simulink model "simulate_fixed_complex_trajectories"  (R2021a)
settings: Solver=VariableStepAuto  StartTime=0.0  StopTime=100  RelTol=1e-3
PreLoadFcn:
  | set_param_fixed_complex;
undefined symbols (not defined in the file or in its folder): ParamFixComplex, ParamFixLine, ParamFixOrb
settings Model: Creator=diogo  LastModifiedBy=Nunes
settings SolverCC: AlgebraicLoopSolver=TrustRegion
settings DebuggingCC: SFMachineParentedDataDiag=warning

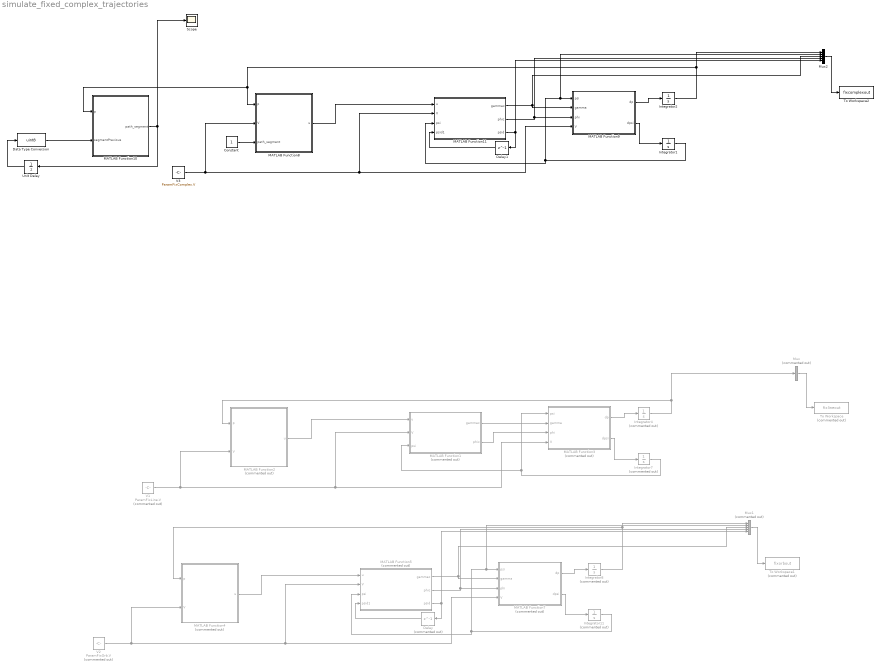
== system simulate_fixed_complex_trajectories ==
  Constant : Constant  OutDataTypeStr=uint8
  Data Type Conversion : DataTypeConversion  OutDataTypeStr=uint8
  Delay : Delay  Commented=on  DelayLength=1  InitialCondition=0
  Delay1 : Delay  DelayLength=1  InitialCondition=0
  Integrator1 : Integrator  InitialCondition=ParamFixComplex.psi0
  Integrator11 : Integrator  Commented=on  InitialCondition=ParamFixOrb.psi0
  Integrator2 : Integrator  InitialCondition=ParamFixComplex.p0
  Integrator4 : Integrator  Commented=on  InitialCondition=ParamFixLine.p0
  Integrator7 : Integrator  Commented=on  InitialCondition=ParamFixLine.psi0
  Integrator8 : Integrator  Commented=on  InitialCondition=ParamFixOrb.p0
  MATLAB Function1 : MATLAB Function  Commented=on  TreatAsAtomicUnit=on
  MATLAB Function10 : MATLAB Function  TreatAsAtomicUnit=on
  MATLAB Function11 : MATLAB Function  TreatAsAtomicUnit=on
  MATLAB Function2 : MATLAB Function  Commented=on  TreatAsAtomicUnit=on
  MATLAB Function3 : MATLAB Function  Commented=on  TreatAsAtomicUnit=on
  MATLAB Function4 : MATLAB Function  Commented=on  TreatAsAtomicUnit=on
  MATLAB Function5 : MATLAB Function  Commented=on  TreatAsAtomicUnit=on
  MATLAB Function7 : MATLAB Function  Commented=on  TreatAsAtomicUnit=on
  MATLAB Function8 : MATLAB Function  TreatAsAtomicUnit=on
  MATLAB Function9 : MATLAB Function  TreatAsAtomicUnit=on
  Mux : Mux  Commented=on  Inputs=1
  Mux1 : Mux  Commented=on  Inputs=5
  Mux2 : Mux  Inputs=5
  Scope : Scope
  To Workspace : ToWorkspace  Commented=on  VariableName=fixlineout  SaveFormat=Timeseries  SampleTime=-1
  To Workspace1 : ToWorkspace  Commented=on  VariableName=fixorbout  SaveFormat=Timeseries  SampleTime=-1
  To Workspace2 : ToWorkspace  VariableName=fixcomplexout  SaveFormat=Timeseries  SampleTime=-1
  Unit Delay : UnitDelay  InitialCondition=1  SampleTime=-1  HasFrameUpgradeWarning=on
  V1 : Constant  Commented=on  Value=ParamFixLine.V
  V2 : Constant  Commented=on  Value=ParamFixOrb.V
  V3 : Constant  Value=ParamFixComplex.V
  wires:
  MATLAB Function3/1(dp) -> Integrator4/1
  MATLAB Function3/2(dpsi) -> Integrator7/1
  Integrator7/1 -> MATLAB Function1/3(psi), MATLAB Function3/1(psi)
  MATLAB Function1/2(phic) -> MATLAB Function3/3(phi)
  MATLAB Function1/1(gammac) -> MATLAB Function3/2(gamma)
  V1/1 -> MATLAB Function2/2(V), MATLAB Function1/2(V), MATLAB Function3/4(V)
  Integrator4/1 -> MATLAB Function2/1(p), Mux/1
  MATLAB Function2/1(u) -> MATLAB Function1/1(u)
  Mux/1 -> To Workspace/1
  MATLAB Function5/2(phic) -> Mux1/4, MATLAB Function7/3(phi)
  MATLAB Function7/1(dp) -> Integrator8/1
  V2/1 -> MATLAB Function4/2(V), MATLAB Function5/2(V), MATLAB Function7/4(V)
  MATLAB Function7/2(dpsi) -> Integrator11/1
  Integrator11/1 -> Mux1/2, MATLAB Function7/1(psi), MATLAB Function5/3(psi)
  Mux1/1 -> To Workspace1/1
  MATLAB Function5/1(gammac) -> Mux1/3, MATLAB Function7/2(gamma)
  Integrator8/1 -> MATLAB Function4/1(p), Mux1/1
  MATLAB Function4/1(u) -> MATLAB Function5/1(u)
  MATLAB Function5/3(psid) -> Mux1/5, Delay/1
  Delay/1 -> MATLAB Function5/4(psid1)
  MATLAB Function11/3(psid) -> Mux2/5, Delay1/1
  Delay1/1 -> MATLAB Function11/4(psid1)
  V3/1 -> MATLAB Function8/2(V), MATLAB Function11/2(V), MATLAB Function9/4(V)
  Integrator2/1 -> Mux2/1, MATLAB Function8/1(p), MATLAB Function10/1(p)
  MATLAB Function11/1(gammac) -> Mux2/3, MATLAB Function9/2(gamma)
  Mux2/1 -> To Workspace2/1
  MATLAB Function8/1(u) -> MATLAB Function11/1(u)
  MATLAB Function9/1(dp) -> Integrator2/1
  MATLAB Function9/2(dpsi) -> Integrator1/1
  MATLAB Function11/2(phic) -> Mux2/4, MATLAB Function9/3(phi)
  Integrator1/1 -> MATLAB Function11/3(psi), Mux2/2, MATLAB Function9/1(psi)
  Unit Delay/1 -> Data Type Conversion/1
  Data Type Conversion/1 -> MATLAB Function10/2(segmentPrevious)
  MATLAB Function10/1(path_segment) -> Scope/1, Unit Delay/1
  Constant/1 -> MATLAB Function8/3(path_segment)

== matlab function simulate_fixed_complex_trajectories/MATLAB Function10 ==
  data: p input; path_segment output; ParamFixComplex parameter; segmentPrevious input
function path_segment   = complex_path_manager(p,  ParamFixComplex, segmentPrevious)
 
path_segment = segmentPrevious;

number_of_segments = size(ParamFixComplex.c0_l);
number_of_segments = number_of_segments(2);

if path_segment == number_of_segments
    
   % number_of_segments = cast(number_of_segments, "uint8");
    %segment = number_of_segments - 1;

    
    c_n = ParamFixComplex.c0_l(1, path_segment );   
    c_e = ParamFixComplex.c0_l(2,path_segment );
    c_d = ParamFixComplex.c0_l(3,path_segment);

else 
    
    c_n = ParamFixComplex.c0_l(1, path_segment + 1);   
    c_e = ParamFixComplex.c0_l(2,path_segment + 1);
    c_d = ParamFixComplex.c0_l(3,path_segment + 1);

end



distance_to_next_path = sqrt((c_n - p(1))^2 + (c_e - p(2))^2 + (c_d - p(3))^2);
proximity_radius = 10;


if distance_to_next_path < proximity_radius
    path_segment = path_segment + 1 ;

end







end


















% if distance_to_next_path < proximity_radius
%     segment = 2;

% %second line starting point
% c_n = ParamFixComplex.c0_l(1, segmentPrevious + 1);   
% c_e = ParamFixComplex.c0_l(2,segmentPrevious + 1);
% c_d = ParamFixComplex.c0_l(3,segmentPrevious + 1);
% 
% 
% distance_to_next_path = sqrt((c_n - p(1))^2 + (c_e - p(2))^2 + (c_d - p(3))^2);
% proximity_radius = 10;
% 
% 
% if distance_to_next_path < proximity_radius
%     segment = 2;
% 
% else 
%     segment = segmentPrevious;
% end
% 
% % path_segment = segment;

== matlab function simulate_fixed_complex_trajectories/MATLAB Function11 ==
  data: u input; V input; psi input; psid1 input; gammac output; phic output; ParamFixComplex parameter; psid output
function [  gammac, phic, psid] = path_following_controller(u, V, psi, psid1, ParamFixComplex)

gamma_limit = ParamFixComplex.gamma_limit;
phi_limit = ParamFixComplex.phi_limit;
kphi = ParamFixComplex.kphi;

gammac = -sat(asin(u(3)/V), gamma_limit);

psid = atan2(u(2),u(1));

while abs(psid - psid1) > 3*pi/2
    if((psid - psid1) > 3*pi/2) 
        psid = psid- 2*pi;
    elseif ((psid - psid1) < - 3*pi/2)
        psid = psid + 2*pi;
    end
end

if(abs(psid - psid1) > pi)
    xpto = 0;
end;

phic = sat(kphi*(psid - psi), phi_limit);

end

== matlab function simulate_fixed_complex_trajectories/MATLAB Function1 ==
  data: u input; V input; psi input; gammac output; phic output; ParamFixLine parameter
function [  gammac, phic] = path_following_controller(u, V, psi, ParamFixLine)


gamma_limit = ParamFixLine.gamma_limit;
phi_limit = ParamFixLine.phi_limit;
kphi = ParamFixLine.kphi;

gammac = -sat(asin(u(3)/V), gamma_limit);

psid = atan2(u(2),u(1));

phic = sat(kphi*(psid- psi), phi_limit);

end

== matlab function simulate_fixed_complex_trajectories/MATLAB Function2 ==
  data: p input; u output; V input; ParamFixLine parameter
function u  = straight_path_generator(p, V, ParamFixLine)


%Variables

psi_l = ParamFixLine.psi_l;  %desired heading angle
gamma_l = ParamFixLine.gamma_l; %desired flight path angle

c_n = ParamFixLine.c0(1);    %path starting point
c_e = ParamFixLine.c0(2);
c_d = ParamFixLine.c0(3);

r_n = p(1);    %position
r_e = p(2);
r_d = p(3);
r = [r_n; r_e; r_d];

cl = [c_n; c_e; c_d];

ql = [cos(psi_l)*cos(gamma_l) ; sin(psi_l)*cos(gamma_l) ; -sin(gamma_l) ];
%direction of line




n_lon = [ -sin(psi_l) ; cos(psi_l) ; 0 ]; 

n_lat = [-cos(psi_l)*sin(gamma_l) ; -sin(psi_l)*sin(gamma_l) ; -cos(gamma_l) ];

k1 = 1;
k2 = 1;

%u_line = k1*(n_lon*transpose(n_lon) +  n_lat*transpose(n_lat))*(r - cl) + k2*cross(n_lon,n_lat);
u_line = -k1*(n_lon*n_lon' +  n_lat*n_lat')*(r - cl) - k2*cross(n_lon,n_lat);

u = V*(u_line/norm(u_line));



end

== matlab function simulate_fixed_complex_trajectories/MATLAB Function3 ==
  data: psi input; gamma input; phi input; V input; dp output; dpsi output
function [dp, dpsi] = drone_model(psi,gamma,phi, V)
    
    %criar param para generalizar os valores
    
    %dp = [V*cos(psi)*cos(gamma); V*sin(psi)*cos(gamma); -V*sin(gamma)]
    
    dpn =V*cos(psi)*cos(gamma);
    dpe = V*sin(psi)*cos(gamma);
    dpd = -V*sin(gamma);
    dpsi =  (9.8/V)*tan(phi);
    
    dp = [dpn; dpe; dpd];
end

== matlab function simulate_fixed_complex_trajectories/MATLAB Function4 ==
  data: p input; u output; V input; ParamFixOrb parameter
function u  = orbit_path_generator(p, V, ParamFixOrb)


%Variables

 Rh = ParamFixOrb.Rh;
 lambda = ParamFixOrb.lambda;
 gamma_h = ParamFixOrb.gamma_h;
 psi_h = ParamFixOrb.psi_h;
 
k1 = ParamFixOrb.k1;
k2 = ParamFixOrb.k2;
 

ch = ParamFixOrb.ch;

c_n = ch(1);    %center of helix
c_e = ch(2);
c_d = ch(3);


 r_n = p(1);
 r_e = p(2);
 r_d = p(3);
 
 
%r0 = ch + [Rh*cos(psi_h) ; Rh*sin(psi_h) ; 0];

dalpha_cyl = transpose( [ 2*(r_n - c_n)/Rh ; 2*(r_e - c_e)/Rh ; 0 ] );

dalpha_pl = transpose( [ (tan(gamma_h)/lambda)*(-(r_e - c_e))/( (r_n - c_n)^2 + (r_e - c_e)^2 ) ; (tan(gamma_h)/lambda)*(r_n - c_e)/( (r_n - c_n)^2 + (r_e - c_e)^2 )  ; 1/Rh ] );


alpha_cyl = ( (r_n - c_n)/Rh )^2 + ( (r_e - c_e)/Rh )^2 -1;

alpha_pl = ( (r_d - c_d)/Rh )^2 + (tan(gamma_h)/lambda)*(atan( (r_e - c_e)/(r_n - c_n) ) - psi_h);

u_line = k1*(-alpha_cyl*dalpha_cyl + alpha_pl*dalpha_pl) + lambda*k2*( (2/Rh)*transpose([ (r_e - c_e)/Rh ; -(r_n - c_n)/Rh ; lambda*tan(gamma_h) ]) );

u =  V*(u_line/norm(u_line));





end

== matlab function simulate_fixed_complex_trajectories/MATLAB Function5 ==
  data: u input; V input; psi input; psid1 input; gammac output; phic output; ParamFixOrb parameter; psid output
function [  gammac, phic, psid] = path_following_controller(u, V, psi, psid1, ParamFixOrb)

gamma_limit = ParamFixOrb.gamma_limit;
phi_limit = ParamFixOrb.phi_limit;
kphi = ParamFixOrb.kphi;

gammac = -sat(asin(u(3)/V), gamma_limit);

psid = atan2(u(2),u(1));

while abs(psid - psid1) > 3*pi/2
    if((psid - psid1) > 3*pi/2) 
        psid = psid- 2*pi;
    elseif ((psid - psid1) < - 3*pi/2)
        psid = psid + 2*pi;
    end
end

if(abs(psid - psid1) > pi)
    xpto = 0;
end;

phic = sat(kphi*(psid - psi), phi_limit);

end

== matlab function simulate_fixed_complex_trajectories/MATLAB Function8 ==
  data: p input; u output; V input; ParamFixComplex parameter; path_segment input
function u  = complex_path_generator(p, V, ParamFixComplex, path_segment)


%Variables

psi_l = ParamFixComplex.psi_l(path_segment);  %desired heading angle
gamma_l = ParamFixComplex.gamma_l(path_segment); %desired flight path angle

c_n = ParamFixComplex.c0_l(1,path_segment);    %path starting point
c_e = ParamFixComplex.c0_l(2,path_segment);
c_d = ParamFixComplex.c0_l(3,path_segment);


% 
% psi_l = ParamFixComplex.psi_l(path_segment);  %desired heading angle
% gamma_l = ParamFixComplex.gamma_l(path_segment); %desired flight path angle
% 
% c_n = ParamFixComplex.c0_l(1,path_segment);    %path starting point
% c_e = ParamFixComplex.c0_l(2,path_segment);
% c_d = ParamFixComplex.c0_l(3,path_segment);
% 
% 





r_n = p(1);    %position
r_e = p(2);
r_d = p(3);
r = [r_n; r_e; r_d];

cl = [c_n; c_e; c_d];





n_lon = [ -sin(psi_l) ; cos(psi_l) ; 0 ]; 

n_lat = [-cos(psi_l)*sin(gamma_l) ; -sin(psi_l)*sin(gamma_l) ; -cos(gamma_l) ];

k1 = 1;
k2 = 1;

%u_line = k1*(n_lon*transpose(n_lon) +  n_lat*transpose(n_lat))*(r - cl) + k2*cross(n_lon,n_lat);
u_line = -k1*(n_lon*n_lon' +  n_lat*n_lat')*(r - cl) - k2*cross(n_lon,n_lat);

u = V*(u_line/norm(u_line));





















%ORB
% %Variables
% 
%  Rh = ParamFixOrb.Rh;
%  lambda = ParamFixOrb.lambda;
%  gamma_h = ParamFixOrb.gamma_h;
%  psi_h = ParamFixOrb.psi_h;
%  
% k1 = ParamFixOrb.k1;
% k2 = ParamFixOrb.k2;
%  
% 
% ch = ParamFixOrb.ch;
% 
% c_n = ch(1);    %center of helix
% c_e = ch(2);
% c_d = ch(3);
% 
% 
%  r_n = p(1);
%  r_e = p(2);
%  r_d = p(3);
%  
%  
% %r0 = ch + [Rh*cos(psi_h) ; Rh*sin(psi_h) ; 0];
% 
% dalpha_cyl = transpose( [ 2*(r_n - c_n)/Rh ; 2*(r_e - c_e)/Rh ; 0 ] );
% 
% dalpha_pl = transpose( [ (tan(gamma_h)/lambda)*(-(r_e - c_e))/( (r_n - c_n)^2 + (r_e - c_e)^2 ) ; (tan(gamma_h)/lambda)*(r_n - c_e)/( (r_n - c_n)^2 + (r_e - c_e)^2 )  ; 1/Rh ] );
% 
% 
% alpha_cyl = ( (r_n - c_n)/Rh )^2 + ( (r_e - c_e)/Rh )^2 -1;
% 
% alpha_pl = ( (r_d - c_d)/Rh )^2 + (tan(gamma_h)/lambda)*(atan( (r_e - c_e)/(r_n - c_n) ) - psi_h);
% 
% u_line = k1*(-alpha_cyl*dalpha_cyl + alpha_pl*dalpha_pl) + lambda*k2*( (2/Rh)*transpose([ (r_e - c_e)/Rh ; -(r_n - c_n)/Rh ; lambda*tan(gamma_h) ]) );
% 
% u =  V*(u_line/norm(u_line));



end

== matlab function simulate_fixed_complex_trajectories/MATLAB Function7 ==
  data: psi input; gamma input; phi input; V input; dp output; dpsi output
function [dp,dpsi] = drone_model(psi,gamma,phi, V)
    
    %criar param para generalizar os valores
    
    %dp = [V*cos(psi)*cos(gamma); V*sin(psi)*cos(gamma); -V*sin(gamma)]
    
    dpn =V*cos(psi)*cos(gamma);
    dpe = V*sin(psi)*cos(gamma);
    dpd = -V*sin(gamma);
    dpsi =  (9.8/V)*tan(phi);
    
    dp = [dpn; dpe; dpd];
    
end

== matlab function simulate_fixed_complex_trajectories/MATLAB Function9 ==
  data: psi input; gamma input; phi input; V input; dp output; dpsi output
function [dp,dpsi] = drone_model(psi,gamma,phi, V)
    
    %criar param para generalizar os valores
    
    %dp = [V*cos(psi)*cos(gamma); V*sin(psi)*cos(gamma); -V*sin(gamma)]
    
    dpn =V*cos(psi)*cos(gamma);
    dpe = V*sin(psi)*cos(gamma);
    dpd = -V*sin(gamma);
    dpsi =  (9.8/V)*tan(phi);
    
    dp = [dpn; dpe; dpd];
    
end
